simulink model "Template_PID_model"  (R2021a)
settings: Solver=VariableStepAuto  StartTime=0.0  StopTime=10.0  RelTol=1e-3
settings Model: Creator=Intuito_PC  LastModifiedBy=Intuito_PC

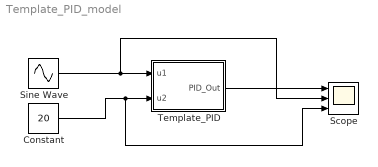
== system Template_PID_model ==
  Constant : Constant  Value=20
  Scope : Scope  NumInputPorts=3
  Sine Wave : Sin  Amplitude=25  SampleTime=0
  Template_PID : MATLAB Function  TreatAsAtomicUnit=on
  wires:
  Sine Wave/1 -> Scope/2, Template_PID/1(u1)
  Constant/1 -> Scope/3, Template_PID/2(u2)
  Template_PID/1(PID_Out) -> Scope/1

== matlab function Template_PID_model/Template_PID ==
  data: u1 input; PID_Out output; u2 input
function PID_Out = fcn(u1, u2)
% PID Constants
kP = 0.1; %Proportinal Constant
kI = 2;  %Integral Constant
kD = 0.5;  %Differential Constant
% Compute PID Control
PIDdiff = (u2 - u1);
PIDintegral =+ PIDdiff ;
PID_Out = kP*PIDdiff + kI*PIDintegral;
end
